simulink model "bizhang"  (R2017a)
settings: Solver=VariableStepAuto  StartTime=0.0  StopTime=10.0  RelTol=1e-3  EnableMultiTasking=on
values from neighbouring files (symbols this model uses):
  scan = receive(laser)    [leida.m]
undefined symbols (not defined in the file or in its folder): Angular, Linear
libraries: robotlib x3, simulink x1
settings Model: Creator=Wangkuo  LastModifiedBy=nylyl
settings OptimizationCC: LifeSpan=inf
settings DebuggingCC: SFUnexpectedBacktrackingDiag=warning  SFNoUnconditionalDefaultTransitionDiag=warning  SFExecutionAtInitializationDiag=none
settings GRTTargetCC: TargetLangStandard=C89/C90 (ANSI)  GeneratePreprocessorConditionals=Disable all
settings ConfigComp: CovMetricSettings=dw  CovHtmlReporting=on  CovSaveCumulativeToWorkspaceVar=on  CovSaveSingleToWorkspaceVar=on  CovExternalEMLEnable=off

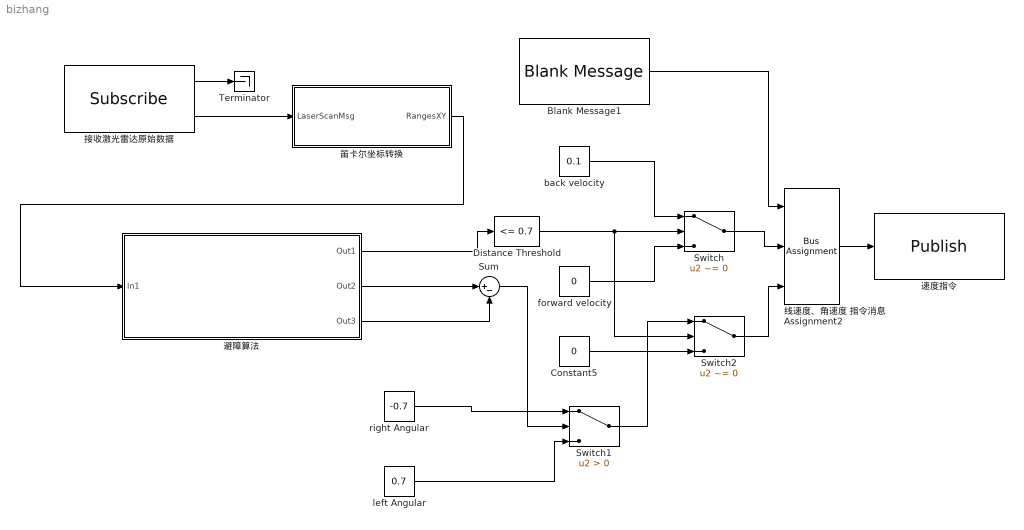
== system bizhang ==
  " left Angular" : Constant  Value=0.7
  Blank Message1 : robotlib/Blank Message  SourceLibraryInfo=This block requires Robotics System Toolbox  messageType=geometry_msgs/Twist  SampleTime=inf
      settings: SourceProductBaseCode=RO
  Constant5 : Constant  Value=0
  Distance Threshold : simulink/Logic and Bit Operations/Compare To Constant  relop=<=  const=0.7  OutDataTypeStr=boolean
  Sum : Sum  Inputs=|+-
  Switch : Switch  Criteria=u2 ~= 0  Threshold=0.7
  Switch1 : Switch  Criteria=u2 > Threshold
  Switch2 : Switch  Criteria=u2 ~= 0
  Terminator : Terminator
  back velocity : Constant  Value=0.1
  forward velocity : Constant  Value=0
  "right Angular " : Constant  Value=-0.7
  接收激光雷达原始数据 : robotlib/Subscribe  SourceLibraryInfo=This block requires Robotics System Toolbox  topicSource=Select from ROS network  topic=/scan  messageType=sensor_msgs/LaserScan  sampleTime=-1  messageQueueLength=1
      settings: SourceProductBaseCode=RO
  笛卡尔坐标转换 : MATLAB Function  TreatAsAtomicUnit=on
  线速度、角速度 指令消息 Assignment2 : BusAssignment  DialogController=Simulink.DDGSource_BusAssignment  AssignedSignals=Linear.X,Angular.Z
  速度指令 : robotlib/Publish  SourceLibraryInfo=This block requires Robotics System Toolbox  topicSource=Select from ROS network  topic=/mobile_base/commands/velocity  messageType=geometry_msgs/Twist  messageQueueLength=105
      settings: SourceProductBaseCode=RO
  避障算法 : Subsystem
      mask Display: disp('避障算法模块');
  wires:
  Blank Message1/1 -> 线速度、角速度 指令消息 Assignment2/1
  线速度、角速度 指令消息 Assignment2/1 -> 速度指令/1
  Switch/1 -> 线速度、角速度 指令消息 Assignment2/2
  Switch1/1 -> Switch2/1
  Constant5/1 -> Switch2/3
  Sum/1 -> Switch1/2
  Switch2/1 -> 线速度、角速度 指令消息 Assignment2/3
  " left Angular"/1 -> Switch1/3
  back velocity/1 -> Switch/1
  forward velocity/1 -> Switch/3
  Distance Threshold/1 -> Switch2/2, Switch/2
  接收激光雷达原始数据/1 -> Terminator/1
  接收激光雷达原始数据/2 -> 笛卡尔坐标转换/1(LaserScanMsg)
  笛卡尔坐标转换/1(RangesXY) -> 避障算法/1(In1)
  避障算法/1(Out1) -> Distance Threshold/1
  避障算法/2(Out2) -> Sum/1
  避障算法/3(Out3) -> Sum/2
  "right Angular "/1 -> Switch1/1

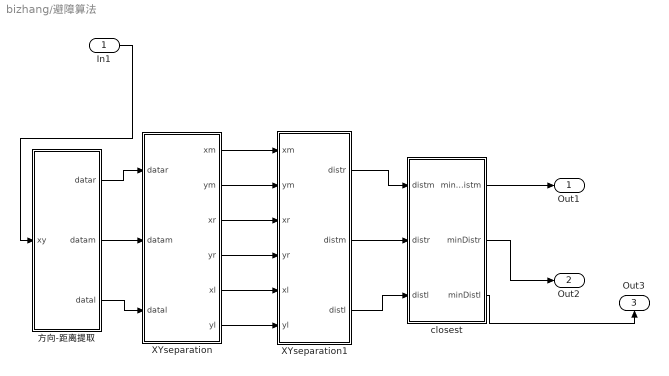
== system bizhang/避障算法 ==
  In1 : Inport
  XYseparation : MATLAB Function  TreatAsAtomicUnit=on
  XYseparation1 : MATLAB Function  TreatAsAtomicUnit=on
  closest : MATLAB Function  TreatAsAtomicUnit=on
  方向-距离提取 : MATLAB Function  TreatAsAtomicUnit=on
  Out1 : Outport
  Out2 : Outport  Port=2
  Out3 : Outport  Port=3
  wires:
  XYseparation1/3(distl) -> closest/3(distl)
  方向-距离提取/1(datar) -> XYseparation/1(datar)
  XYseparation/2(ym) -> XYseparation1/2(ym)
  In1/1 -> 方向-距离提取/1(xy)
  XYseparation1/2(distm) -> closest/2(distr)
  方向-距离提取/3(datal) -> XYseparation/3(datal)
  XYseparation/5(xl) -> XYseparation1/5(xl)
  XYseparation/6(yl) -> XYseparation1/6(yl)
  方向-距离提取/2(datam) -> XYseparation/2(datam)
  XYseparation1/1(distr) -> closest/1(distm)
  XYseparation/3(xr) -> XYseparation1/3(xr)
  XYseparation/1(xm) -> XYseparation1/1(xm)
  XYseparation/4(yr) -> XYseparation1/4(yr)
  closest/2(minDistr) -> Out2/1
  closest/1(minDistm) -> Out1/1
  closest/3(minDistl) -> Out3/1

== matlab function bizhang/避障算法/XYseparation1 ==
  data: distr output; distm output; distl output; xm input; ym input; xr input; yr input; xl input; yl input
function [ distr , distm ,distl]  = XYsepar(xm,ym,xr,yr,xl,yl)
%#codegen

        distr = sqrt(xr.^2 + yr.^2);
      distm = sqrt(xm.^2 + ym.^2);
      distl = sqrt(xl.^2 + yl.^2);
end

== matlab function bizhang/避障算法/方向-距离提取 ==
  data: datar output; datam output; datal output; xy input
function [datar,datam,datal]= cutAngle(xy)
%#codegen

     datar=xy([70:130],[1:2]);      % 选取70°-130°扇形范围对应的矩阵数据
      datam=xy([150:210],[1:2]);     % 选取150°-210°扇形范围对应的矩阵数据
      datal=xy([230:290],[1:2]); 
       
end

== matlab function bizhang/避障算法/XYseparation ==
  data: xm output; ym output; xr output; datar input; yr output; xl output; yl output; datam input; datal input
function [xm,ym,xr,yr,xl,yl]= XYsepar(datar,datam,datal)
%#codegen

      xr = datar(:,1);
      yr = datar(:,2);
       xm = datam(:,1);
       ym=  datam(:,2);
      xl = datal(:,1);
      yl=  datal(:,2);
end

== matlab function bizhang/避障算法/closest ==
  data: distm input; minDistm output; minDistr output; minDistl output; distr input; distl input
function [ minDistm,minDistr,minDistl]   = min(distm,distr,distl)
%#codegen
      minDistm = min(distm);
       minDistr = min(distr);   
       minDistl = min(distl);
end

== matlab function bizhang/笛卡尔坐标转换 ==
  data: LaserScanMsg input; RangesXY output
function RangesXY  = ExtractRangeData(LaserScanMsg)
% 解析距离数据并将极坐标转换成笛卡尔坐标
Ranges = double(LaserScanMsg.Ranges);
RangesXY=readCartesian(Ranges);
end
